simulink model "radarDFT"  (R2013a)
settings: Solver=ode45  StartTime=0.0  StopTime=90  RelTol=1e-3
PostLoadFcn:
  | bps_model_init(gcs);
undefined symbols (not defined in the file): xlipgetpartsetting
libraries: xbsIndex_r4 x69, xps_library x25, mbee4_library x4
(part 1 of 3)
settings Model: Creator=BEEcube  LastModifiedBy=rijesh
settings DataIOCC: SignalLoggingSaveFormat=ModelDataLogs
settings OptimizationCC: InlineParams=on  ExpressionDepthLimit=2147483647
settings DebuggingCC: FcnCallInpInsideContextMsg=UseLocalSettings
settings GRTTargetCC: CombineOutputUpdateFcns=off  GRTInterface=on

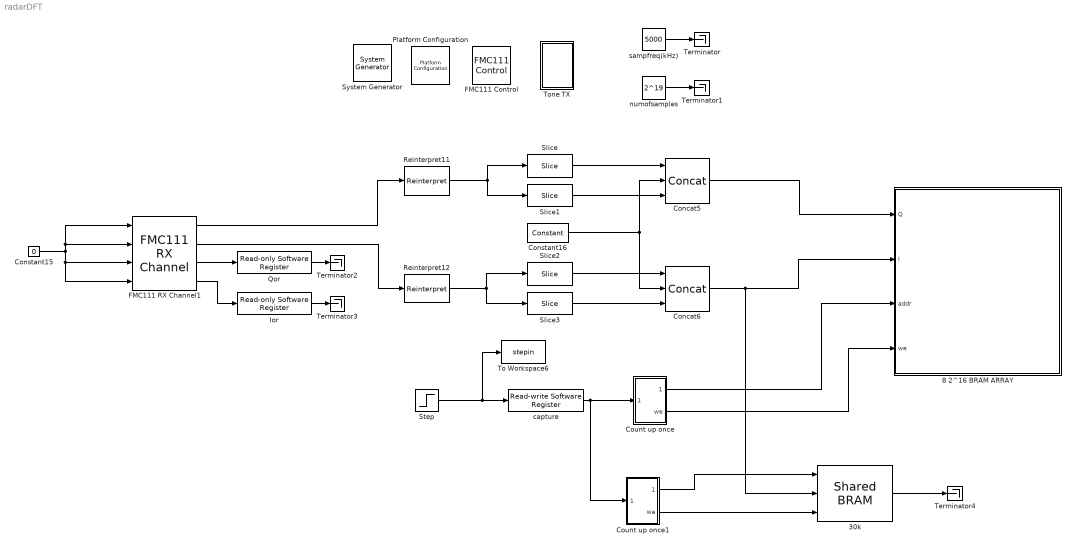
== system radarDFT ==
  " Platform Configuration " : mbee4_library/ Platform Configuration   Tag=xps:xsg,ver:4.5  xsg_ver=14.7  hw_sys=mBEE4  fpga_type=xc6vsx475t  fpga_device='xc6vsx475t-2ff1759'  bp_override=off  bp_choice='mBEE4'  bp_option=base  clk_src=fmc_clk1_fx: User defined clock based on FMC_HPC_CLK1  clk_rate=250000000  ref_clk_rate=250000000  enable_half_rate=off  sample_period=1  update=off
  " System Generator" : xbsIndex_r4/ System Generator  Tag=genX  xilinxfamily=virtex6  part=xc6vsx475t  speed=-2  package=ff1759  synthesis_tool=XST  clock_wrapper=Clock Enables  directory=./radarDFT/sysgen  proj_type=Project Navigator  Synth_file=XST Defaults  Impl_file=ISE Defaults  testbench=off  simulink_period=1  sysclk_period=4  dcm_input_clock_period=10  incr_netlist=off  trim_vbits=Everywhere in SubSystem  dbl_ovrd=According to Block Masks  core_generation=According to Block Masks  run_coregen=off  deprecated_control=off  eval_field=0  block_type=sysgen
  30k : xps_library/Shared BRAM  Tag=xps:bram  arith_type=Unsigned  addr_width=11  bitwidth=32  bin_pt=0  init_vals=0  sample_period=1  update=off
  8 2^16 BRAM ARRAY : Subsystem
  Concat5 : xbsIndex_r4/Concat  num_inputs=3  dbl_ovrd=off  block_type=concat
  Concat6 : xbsIndex_r4/Concat  num_inputs=3  dbl_ovrd=off  block_type=concat
  Constant15 : Constant  Value=0  SampleTime=1
  Constant16 : xbsIndex_r4/Constant  const=0  gui_display_data_type=Fixed-point  arith_type=Unsigned  n_bits=18  bin_pt=0  preci_type=Single  exp_width=8  frac_width=24  explicit_period=off  period=1  equ=P=C  opselect=C  inp2=PCIN>>17  opr=+  inp1=P  carry=CIN  dbl_ovrd=off  block_type=constant
  Count up once : Subsystem
  Count up once1 : Subsystem
  FMC111 Control : mbee4_library/FMC111 Control  Tag=xps:fmc111_ctrl  board_type=FMC111  sample_period=1  update=off
  FMC111 RX Channel1 : mbee4_library/FMC111 RX Channel  Tag=xps:fmc111_rx  channel_number=1  arith_type=Signed  bitwidth=14  bin_pt=0  sample_period=1  update=off
  Ior : xps_library/Read-only Software Register  Tag=xps:sw_reg  io_dir=To Processor  use_strobe=off  arith_type=Unsigned  bitwidth=32  bin_pt=0  sample_period=1  update=off
  Qor : xps_library/Read-only Software Register  Tag=xps:sw_reg  io_dir=To Processor  use_strobe=off  arith_type=Unsigned  bitwidth=32  bin_pt=0  sample_period=1  update=off
  Reinterpret11 : xbsIndex_r4/Reinterpret  force_arith_type=on  arith_type=Unsigned  force_bin_pt=off  bin_pt=0  block_type=reinterpret
  Reinterpret12 : xbsIndex_r4/Reinterpret  force_arith_type=on  arith_type=Unsigned  force_bin_pt=off  bin_pt=0  block_type=reinterpret
  Slice : xbsIndex_r4/Slice  nbits=1  boolean_output=off  mode=Upper Bit Location + Width  bit1=0  base1=MSB of Input  bit0=0  base0=LSB of Input  dbl_ovrd=off  block_type=slice
  Slice1 : xbsIndex_r4/Slice  nbits=13  boolean_output=off  mode=Lower Bit Location + Width  bit1=0  base1=MSB of Input  bit0=0  base0=LSB of Input  dbl_ovrd=off  block_type=slice
  Slice2 : xbsIndex_r4/Slice  nbits=1  boolean_output=off  mode=Upper Bit Location + Width  bit1=0  base1=MSB of Input  bit0=0  base0=LSB of Input  dbl_ovrd=off  block_type=slice
  Slice3 : xbsIndex_r4/Slice  nbits=13  boolean_output=off  mode=Lower Bit Location + Width  bit1=0  base1=MSB of Input  bit0=0  base0=LSB of Input  dbl_ovrd=off  block_type=slice
  Step : Step  SampleTime=1
  Terminator{,1..4} (5 alike) : Terminator
  To Workspace6 : ToWorkspace  VariableName=stepin  SampleTime=-1
  Tone TX : Subsystem  VariantControl=Variant1
  capture : xps_library/Read-write Software Register  Tag=xps:sw_reg  io_dir=From Processor  use_strobe=off  arith_type=Unsigned  bitwidth=32  bin_pt=0  sample_period=1  update=off
  numofsamples : Constant  Value=2^19
  sampfreq(kHz) : Constant  Value=5000
  wires:
  Step/1 -> capture/1, To Workspace6/1
  Constant15/1 -> FMC111 RX Channel1/1, FMC111 RX Channel1/2, FMC111 RX Channel1/4, FMC111 RX Channel1/3
  FMC111 RX Channel1/3 -> Qor/1
  FMC111 RX Channel1/4 -> Ior/1
  FMC111 RX Channel1/1 -> Reinterpret11/1
  FMC111 RX Channel1/2 -> Reinterpret12/1
  Reinterpret11/1 -> Slice1/1, Slice/1
  Reinterpret12/1 -> Slice2/1, Slice3/1
  Constant16/1 -> Concat5/2, Concat6/2
  Concat5/1 -> 8 2^16 BRAM ARRAY/1(Q)
  sampfreq(kHz)/1 -> Terminator/1
  numofsamples/1 -> Terminator1/1
  capture/1 -> Count up once1/1(start), Count up once/1(start)
  Count up once/1(addr) -> 8 2^16 BRAM ARRAY/3(addr)
  Count up once/2(we) -> 8 2^16 BRAM ARRAY/4(we)
  Slice/1 -> Concat5/1
  Slice1/1 -> Concat5/3
  Slice3/1 -> Concat6/3
  Slice2/1 -> Concat6/1
  Qor/1 -> Terminator2/1
  Ior/1 -> Terminator3/1
  30k/1 -> Terminator4/1
  Count up once1/2(we) -> 30k/3
  Count up once1/1(addr) -> 30k/1
  Concat6/1 -> 30k/2, 8 2^16 BRAM ARRAY/2(I)
